simulink model "mpc_payload"  (R2020a)
settings: Solver=ode3  StartTime=0.0  StopTime=200  FixedStep=Ts_sim  RelTol=1e-3
InitFcn:
  | initialise_ros_iris_payload
values from neighbouring files (symbols this model uses):
  A_mpc = A_havok    [initialize_mpc_iris_no_load.m]    (also in initialize_mpc_iris_payload.m = [zeros( size(A_mpc,1), num_axis ), A_mpc])
  enable_mpc_control = 1    [initialise_ros_iris_payload.m]
  max_vel_xy = 5    [initialise_iris_gains.m]
  max_vel_z_down = 5    [initialise_iris_gains.m]
  max_vel_z_up = 5    [initialise_iris_gains.m]
  mpc_step_time = 2    [initialise_ros_iris_payload.m]
  MPC_XY_VEL_D_ACC = 0.2    [initialise_iris_gains.m]
  MPC_XY_VEL_I_ACC = 0.4    [initialise_iris_gains.m]
  MPC_XY_VEL_P_ACC = 1.8    [initialise_iris_gains.m]
  MPC_Z_VEL_D_ACC = 0    [initialise_iris_gains.m]
  MPC_Z_VEL_I_ACC = 2    [initialise_iris_gains.m]
  MPC_Z_VEL_P_ACC = 4    [initialise_iris_gains.m]
  Ts_pos_control = 0.01    [initialise_ros_iris_payload.m]
  vel_step_size = 1    [initialise_ros_iris_payload.m]
  y_ext_0 = zeros(q*ny, 1)    [initialize_mpc_iris_no_load.m]    (also in initialize_mpc_iris_payload.m)
undefined symbols (not defined in the file or in its folder): DiscIntNeverNeededParam, MPC_ACC_DOWN_MAX, MPC_ACC_HOR_MAX, MPC_ACC_UP_MAX, ny, q, q_int_lim, u_bar, vel_filt_denom, vel_filt_num, X, Y, Z
libraries: robotlib x6, simulink x3, robotgazebolib x1, mpclib x1
settings Model: Creator=esl  LastModifiedBy=murray
settings SolverCC: MinimalZcImpactIntegration=on
settings OptimizationCC: DefaultParameterBehavior=Inlined  GainParamInheritBuiltInType=on  UseFloatMulNetSlope=on  InlineInvariantSignals=on  EnhancedBackFolding=on  PassReuseOutputArgsAs=Individual arguments  ZeroExternalMemoryAtStartup=off  ZeroInternalMemoryAtStartup=off  EfficientFloat2IntCast=on  MaxStackSize=64  OptimizeBlockOrder=speed  DifferentSizesBufferReuse=on  OptimizationCustomize=off  EfficientTunableParamExpr=on
settings DebuggingCC: ReadBeforeWriteMsg=DisableAll  WriteAfterWriteMsg=DisableAll  WriteAfterReadMsg=DisableAll  MultiTaskDSMMsg=none  ParameterTunabilityLossMsg=error  SFMachineParentedDataDiag=error
settings HardwareCC: ProdBitPerPointer=32  ProdBitPerSizeT=32  ProdBitPerPtrDiffT=32  ProdLargestAtomicInteger=Long  ProdLargestAtomicFloat=Double  ProdWordSize=32  ProdHWDeviceType=ARM Compatible->ARM Cortex  UseEmbeddedCoderFeatures=off
settings ModelReferenceCC: UpdateModelReferenceTargets=IfOutOfDate
settings SFSimCC: SFSimEcho=off  MATLABDynamicMemAlloc=off
settings RTWCC: SystemTargetFile=ert.tlc  HardwareBoard=Robot Operating System (ROS)  TemplateMakefile=ert_default_tmf  Toolchain=Catkin  BuildConfiguration=Faster Runs  TargetLang=C++
settings CodeAppCC: ForceParamTrailComments=on  IgnoreCustomStorageClasses=off  OperatorAnnotations=on  SimulinkDataObjDesc=on  SFDataObjDesc=on  InsertBlockDesc=on
settings ERTTargetCC: SupportNonFinite=off  SupportNonInlinedSFcns=on  ERTCustomFileTemplate=rostime_codertarget_file_process.tlc

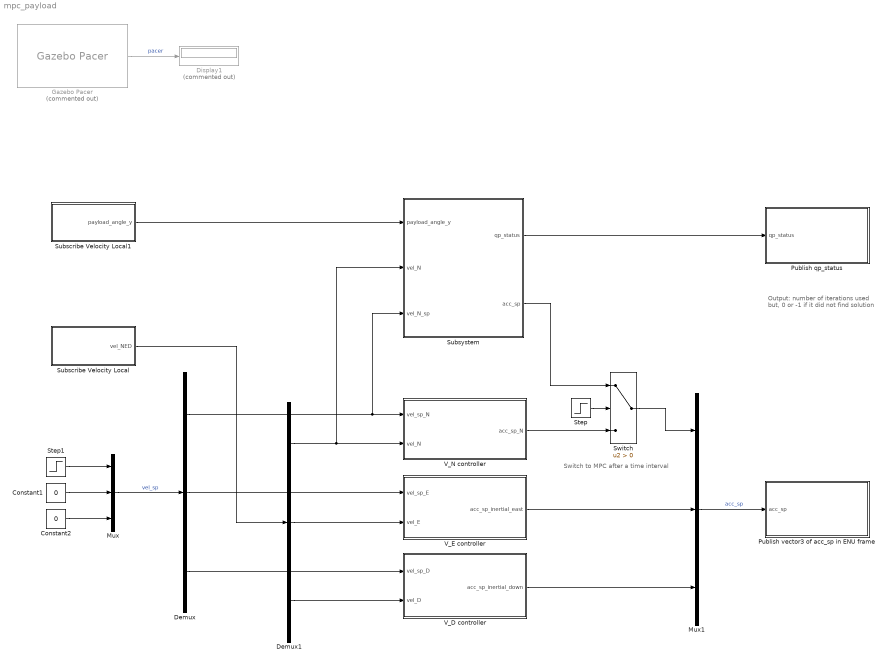
== system mpc_payload ==
  note: Output: number of iterations used
      | but, 0 or -1 if it did not find solution
  note: Switch to MPC after a time interval
  Constant1 : Constant  Value=0
  Constant2 : Constant  Value=0
  Demux : Demux  Outputs=3
  Demux1 : Demux  Outputs=3
  Display1 : Display  Commented=on
  Gazebo Pacer : robotgazebolib/Gazebo Pacer  Commented=on  ResetBehavior=Reset Gazebo simulation time  SampleTime=0.004
      settings: SourceProductBaseCode=RO
  Mux : Mux  Inputs=3
  Mux1 : Mux  Inputs=3
  Publish qp_status : Subsystem
  Publish vector3 of acc_sp in ENU frame : Subsystem
  Step : Step  Time=mpc_step_time  After=enable_mpc_control  SampleTime=0
  Step1 : Step  Time=mpc_step_time  After=vel_step_size  SampleTime=0
  Subscribe Velocity Local : Subsystem
  Subscribe Velocity Local1 : Subsystem
  Subsystem : Subsystem
  Switch : Switch  Criteria=u2 > Threshold
  V_D controller : Subsystem
  V_E controller : Subsystem
  V_N controller : Subsystem
  wires:
  Gazebo Pacer/1 -> Display1/1  "pacer"
  V_D controller/1(acc_sp_inertial_down) -> Mux1/3
  V_E controller/1(acc_sp_inertial_east) -> Mux1/2
  Mux1/1 -> Publish vector3 of acc_sp in ENU frame/1(acc_sp)  "acc_sp"
  Subsystem/2(acc_sp) -> Switch/1
  Mux/1 -> Demux/1  "vel_sp"
  Demux/2 -> V_E controller/1(vel_sp_E)
  Demux/3 -> V_D controller/1(vel_sp_D)
  Demux1/2 -> V_E controller/2(vel_E)
  Demux1/3 -> V_D controller/2(vel_D)
  Subscribe Velocity Local/1(vel_NED) -> Demux1/1
  Demux/1 -> Subsystem/3(vel_N_sp), V_N controller/1(vel_sp_N)
  Demux1/1 -> Subsystem/2(vel_N), V_N controller/2(vel_N)
  Step/1 -> Switch/2
  V_N controller/1(acc_sp_N) -> Switch/3
  Switch/1 -> Mux1/1
  Step1/1 -> Mux/1
  Constant1/1 -> Mux/2
  Constant2/1 -> Mux/3
  Subscribe Velocity Local1/1(payload_angle_y) -> Subsystem/1(payload_angle_y)
  Subsystem/1(qp_status) -> Publish qp_status/1(qp_status)

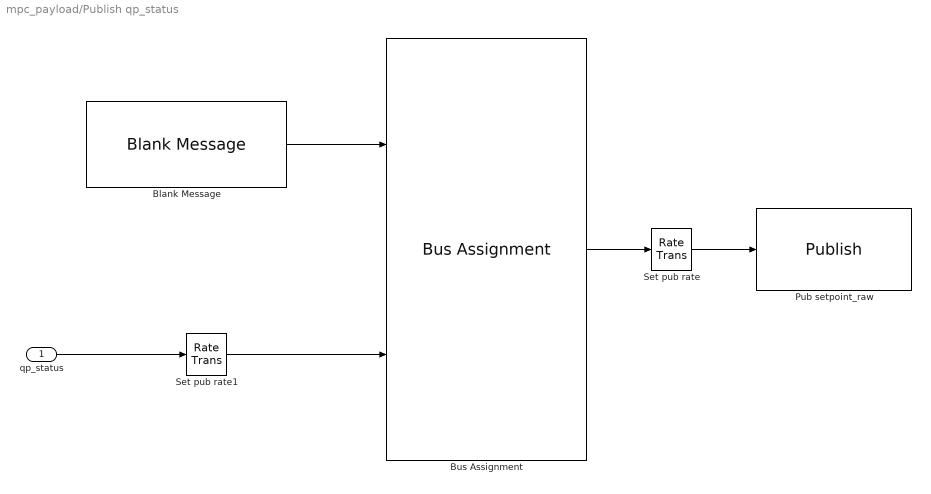
== system mpc_payload/Publish qp_status ==
  qp_status : Inport
  Blank Message : robotlib/Blank Message  messageClass=Message  entityType=std_msgs/Float64  messageType=std_msgs/Float64  SampleTime=inf
  Bus Assignment : BusAssignment  AssignedSignals=Data
  Pub setpoint_raw : robotlib/Publish  topicSource=Specify your own  topic=/simulink/qp_status  messageType=std_msgs/Float64  messageQueueLength=1
  Set pub rate : RateTransition  OutPortSampleTime=Ts_publish
  Set pub rate1 : RateTransition  OutPortSampleTime=Ts_publish
  wires:
  Set pub rate/1 -> Pub setpoint_raw/1
  Bus Assignment/1 -> Set pub rate/1
  Blank Message/1 -> Bus Assignment/1
  qp_status/1 -> Set pub rate1/1
  Set pub rate1/1 -> Bus Assignment/2

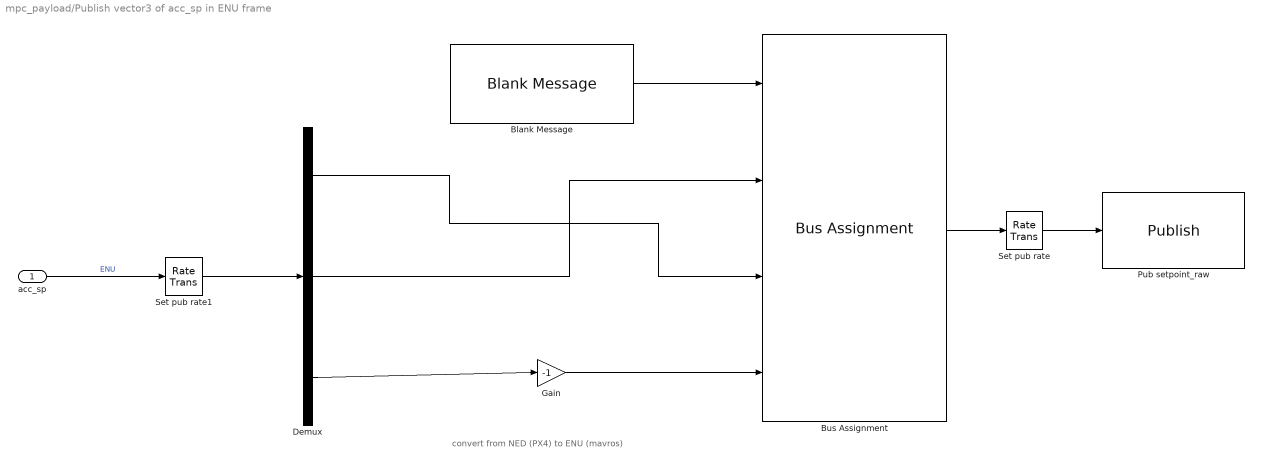
== system mpc_payload/Publish vector3 of acc_sp in ENU frame ==
  note: convert from NED (PX4) to ENU (mavros)
  acc_sp : Inport
  Blank Message : robotlib/Blank Message  messageClass=Message  entityType=geometry_msgs/Vector3  messageType=geometry_msgs/Vector3  SampleTime=inf
  Bus Assignment : BusAssignment  AssignedSignals=X,Y,Z
  Demux : Demux  Outputs=3
  Gain : Gain  Gain=-1
  Pub setpoint_raw : robotlib/Publish  topicSource=Specify your own  topic=/simulink/acc_sp  messageType=geometry_msgs/Vector3  messageQueueLength=1
  Set pub rate : RateTransition  OutPortSampleTime=Ts_publish
  Set pub rate1 : RateTransition  OutPortSampleTime=Ts_publish
  wires:
  Set pub rate/1 -> Pub setpoint_raw/1
  Bus Assignment/1 -> Set pub rate/1
  Blank Message/1 -> Bus Assignment/1
  Demux/1 -> Bus Assignment/3
  Demux/2 -> Bus Assignment/2
  Demux/3 -> Gain/1
  Gain/1 -> Bus Assignment/4
  acc_sp/1 -> Set pub rate1/1  "ENU"
  Set pub rate1/1 -> Demux/1

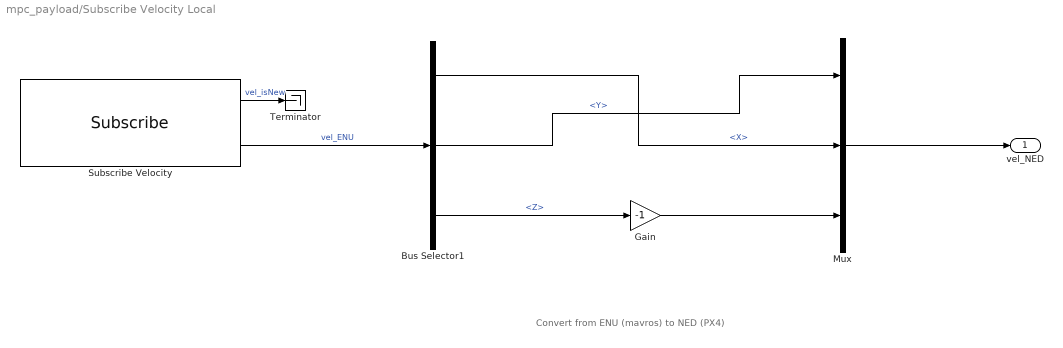
== system mpc_payload/Subscribe Velocity Local ==
  note: Convert from ENU (mavros) to NED (PX4)
  Bus Selector1 : BusSelector  OutputSignals=Twist.Linear.X,Twist.Linear.Y,Twist.Linear.Z
  Gain : Gain  Gain=-1
  Mux : Mux  Inputs=3
  Subscribe Velocity : robotlib/Subscribe  topicSource=Select from ROS network  topic=/mavros/local_position/velocity_local  messageType=geometry_msgs/TwistStamped  sampleTime=Ts_sub  messageQueueLength=1
  Terminator : Terminator
  vel_NED : Outport
  wires:
  Subscribe Velocity/1 -> Terminator/1  "vel_isNew"
  Subscribe Velocity/2 -> Bus Selector1/1  "vel_ENU"
  Mux/1 -> vel_NED/1
  Bus Selector1/1 -> Mux/2  "<X>"
  Bus Selector1/2 -> Mux/1  "<Y>"
  Bus Selector1/3 -> Gain/1  "<Z>"
  Gain/1 -> Mux/3

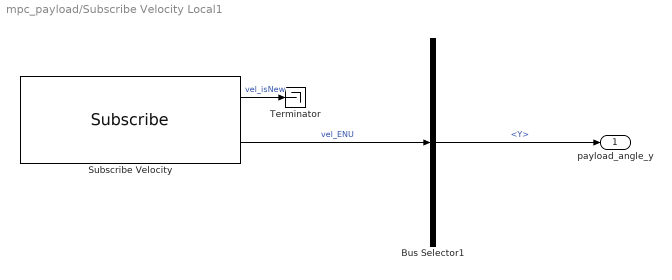
== system mpc_payload/Subscribe Velocity Local1 ==
  Bus Selector1 : BusSelector  OutputSignals=Y
  Subscribe Velocity : robotlib/Subscribe  topicSource=Select from ROS network  topic=/simulink/payload_angles  messageType=geometry_msgs/Vector3  sampleTime=Ts_sub  messageQueueLength=1
  Terminator : Terminator
  payload_angle_y : Outport
  wires:
  Subscribe Velocity/1 -> Terminator/1  "vel_isNew"
  Subscribe Velocity/2 -> Bus Selector1/1  "vel_ENU"
  Bus Selector1/1 -> payload_angle_y/1  "<Y>"

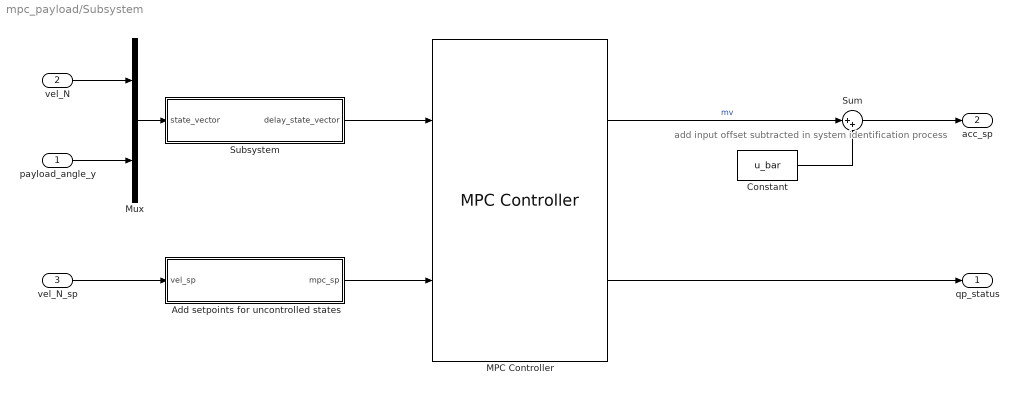
== system mpc_payload/Subsystem ==
  note: add input offset subtracted in system identification process
  payload_angle_y : Inport
  vel_N : Inport  Port=2
  vel_N_sp : Inport  Port=3
  Add setpoints for uncontrolled states : Subsystem
  Constant : Constant  Value=u_bar
  MPC Controller : mpclib/MPC Controller  SCDEnableBlockLinearizationSpecification=on  mpcobj=mpc_iris_payload  is_multiple=0  enable_value=0  return_u0=off  updateMPCinCallerWorkspace=on  md_inport=off  mv_inport=off  uref_inport=off  return_cost=off  return_mvseq=off  return_qpstatus=on  return_xseq=off  return_state=off  return_ovseq=off  state_inport=off  umin_inport=off  umax_inport=off  ymin_inport=off  ymax_inport=off  cc_inport=off  ywt_inport=off  uwt_inport=off  duwt_inport=off  rhoeps_inport=off  pm_inport=off  MaximumP=10  HorizonChoice=FixedHorizon  n_ts=0.03  n_p=166  n_mv=1  n_md=0  n_ud=0  n_mo=140  n_uo=1  BlockDataType=double  SampleTimeInherited=off  switch_inport=off
  Mux : Mux  Inputs=2
  Subsystem : Subsystem
  Sum : Sum  Inputs=|++
  qp_status : Outport  OutDataTypeStr=double  PortDimensions=nu
  acc_sp : Outport  Port=2  OutDataTypeStr=double  PortDimensions=nu
  wires:
  Sum/1 -> acc_sp/1
  MPC Controller/1 -> Sum/1  "mv"
  Constant/1 -> Sum/2
  Subsystem/1(delay_state_vector) -> MPC Controller/1
  Add setpoints for uncontrolled states/1(mpc_sp) -> MPC Controller/2
  vel_N_sp/1 -> Add setpoints for uncontrolled states/1(vel_sp)
  Mux/1 -> Subsystem/1(state_vector)
  vel_N/1 -> Mux/1
  payload_angle_y/1 -> Mux/2
  MPC Controller/2 -> qp_status/1

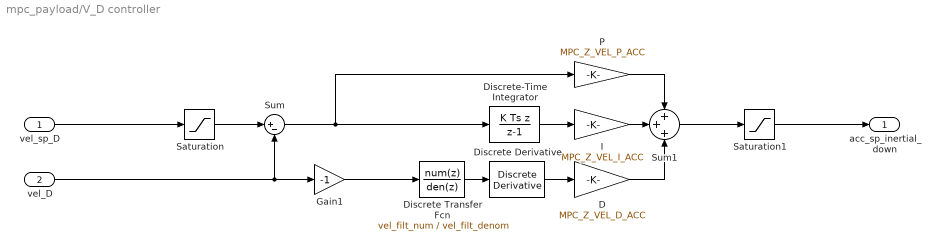
== system mpc_payload/V_D controller ==
  vel_sp_D : Inport  SampleTime=Ts_pos_control
  vel_D : Inport  Port=2  SampleTime=Ts_pos_control
  D : Gain  Gain=MPC_Z_VEL_D_ACC
  Discrete Transfer Fcn : DiscreteTransferFcn  Numerator=vel_filt_num  Denominator=vel_filt_denom
  Discrete Derivative : simulink/Discrete/Discrete Derivative  gainval=1  ICPrevScaledInput=0.0  OutMin=[]  OutMax=[]  OutDataType=fixdt(1, 16)  OutScaling=2^-10  DoSatur=off
  Discrete-Time Integrator : DiscreteIntegrator  IntegratorMethod=Integration: Backward Euler  gainval=1  SampleTime=-1  UpperSaturationLimit=q_int_lim  LowerSaturationLimit=-q_int_lim  ICPrevOutput=DiscIntNeverNeededParam  ICPrevScaledInput=DiscIntNeverNeededParam
  Gain1 : Gain  Gain=-1
  I : Gain  Gain=MPC_Z_VEL_I_ACC
  P : Gain  Gain=MPC_Z_VEL_P_ACC
  Saturation : Saturate  UpperLimit=max_vel_z_up  LowerLimit=-abs(max_vel_z_down)
  Saturation1 : Saturate  UpperLimit=MPC_ACC_UP_MAX  LowerLimit=-MPC_ACC_DOWN_MAX
  Sum : Sum  Inputs=|+-
  Sum1 : Sum  Inputs=+++
  acc_sp_inertial_down : Outport  VectorParamsAs1DForOutWhenUnconnected=off
  wires:
  vel_sp_D/1 -> Saturation/1
  Discrete Derivative/1 -> D/1
  I/1 -> Sum1/2
  D/1 -> Sum1/3
  vel_D/1 -> Gain1/1, Sum/2
  P/1 -> Sum1/1
  Sum/1 -> Discrete-Time Integrator/1, P/1
  Discrete Transfer Fcn/1 -> Discrete Derivative/1
  Saturation/1 -> Sum/1
  Discrete-Time Integrator/1 -> I/1
  Sum1/1 -> Saturation1/1
  Gain1/1 -> Discrete Transfer Fcn/1
  Saturation1/1 -> acc_sp_inertial_down/1

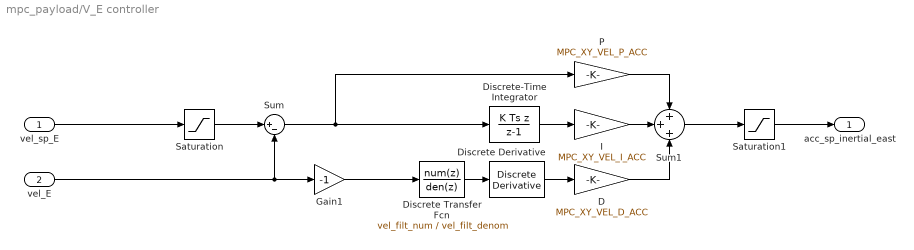
== system mpc_payload/V_E controller ==
  vel_sp_E : Inport  SampleTime=Ts_pos_control
  vel_E : Inport  Port=2  SampleTime=Ts_pos_control
  D : Gain  Gain=MPC_XY_VEL_D_ACC
  Discrete Transfer Fcn : DiscreteTransferFcn  Numerator=vel_filt_num  Denominator=vel_filt_denom
  Discrete Derivative : simulink/Discrete/Discrete Derivative  gainval=1  ICPrevScaledInput=0.0  OutMin=[]  OutMax=[]  OutDataType=fixdt(1, 16)  OutScaling=2^-10  DoSatur=off
  Discrete-Time Integrator : DiscreteIntegrator  IntegratorMethod=Integration: Backward Euler  gainval=1  SampleTime=-1  UpperSaturationLimit=q_int_lim  LowerSaturationLimit=-q_int_lim  ICPrevOutput=DiscIntNeverNeededParam  ICPrevScaledInput=DiscIntNeverNeededParam
  Gain1 : Gain  Gain=-1
  I : Gain  Gain=MPC_XY_VEL_I_ACC
  P : Gain  Gain=MPC_XY_VEL_P_ACC
  Saturation : Saturate  UpperLimit=max_vel_xy  LowerLimit=-max_vel_xy
  Saturation1 : Saturate  UpperLimit=MPC_ACC_HOR_MAX  LowerLimit=-MPC_ACC_HOR_MAX
  Sum : Sum  Inputs=|+-
  Sum1 : Sum  Inputs=+++
  acc_sp_inertial_east : Outport  VectorParamsAs1DForOutWhenUnconnected=off
  wires:
  vel_E/1 -> Gain1/1, Sum/2
  Discrete-Time Integrator/1 -> I/1
  Sum/1 -> Discrete-Time Integrator/1, P/1
  vel_sp_E/1 -> Saturation/1
  Sum1/1 -> Saturation1/1
  Saturation/1 -> Sum/1
  Discrete Transfer Fcn/1 -> Discrete Derivative/1
  Discrete Derivative/1 -> D/1
  I/1 -> Sum1/2
  Gain1/1 -> Discrete Transfer Fcn/1
  P/1 -> Sum1/1
  D/1 -> Sum1/3
  Saturation1/1 -> acc_sp_inertial_east/1

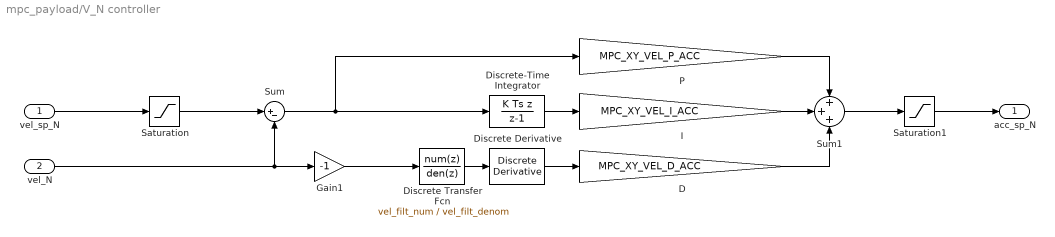
== system mpc_payload/V_N controller ==
  vel_sp_N : Inport  SampleTime=Ts_pos_control
  vel_N : Inport  Port=2  SampleTime=Ts_pos_control
  D : Gain  Gain=MPC_XY_VEL_D_ACC
  Discrete Transfer Fcn : DiscreteTransferFcn  Numerator=vel_filt_num  Denominator=vel_filt_denom
  Discrete Derivative : simulink/Discrete/Discrete Derivative  gainval=1  ICPrevScaledInput=0.0  OutMin=[]  OutMax=[]  OutDataType=fixdt(1, 16)  OutScaling=2^-10  DoSatur=off
  Discrete-Time Integrator : DiscreteIntegrator  IntegratorMethod=Integration: Backward Euler  gainval=1  SampleTime=-1  UpperSaturationLimit=max_vel_xy  LowerSaturationLimit=-max_vel_xy  ICPrevOutput=DiscIntNeverNeededParam  ICPrevScaledInput=DiscIntNeverNeededParam
  Gain1 : Gain  Gain=-1
  I : Gain  Gain=MPC_XY_VEL_I_ACC
  P : Gain  Gain=MPC_XY_VEL_P_ACC
  Saturation : Saturate  UpperLimit=max_vel_xy  LowerLimit=-max_vel_xy
  Saturation1 : Saturate  UpperLimit=MPC_ACC_HOR_MAX  LowerLimit=-MPC_ACC_HOR_MAX
  Sum : Sum  Inputs=|+-
  Sum1 : Sum  Inputs=+++
  acc_sp_N : Outport  VectorParamsAs1DForOutWhenUnconnected=off
  wires:
  vel_N/1 -> Gain1/1, Sum/2
  vel_sp_N/1 -> Saturation/1
  I/1 -> Sum1/2
  Sum/1 -> Discrete-Time Integrator/1, P/1
  P/1 -> Sum1/1
  Sum1/1 -> Saturation1/1
  Discrete Derivative/1 -> D/1
  Discrete Transfer Fcn/1 -> Discrete Derivative/1
  D/1 -> Sum1/3
  Saturation/1 -> Sum/1
  Gain1/1 -> Discrete Transfer Fcn/1
  Discrete-Time Integrator/1 -> I/1
  Saturation1/1 -> acc_sp_N/1

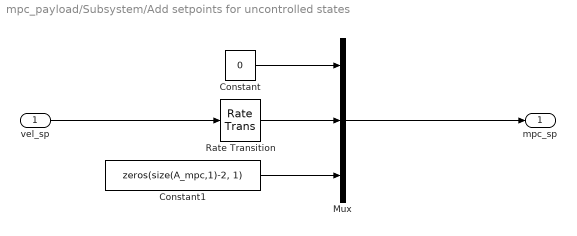
== system mpc_payload/Subsystem/Add setpoints for uncontrolled states ==
  vel_sp : Inport
  Constant : Constant  Value=0
  Constant1 : Constant  Value=zeros(size(A_mpc,1)-2, 1)
  Mux : Mux  Inputs=3
  Rate Transition : RateTransition  Deterministic=off  OutPortSampleTime=Ts_mpc
  mpc_sp : Outport
  wires:
  Constant1/1 -> Mux/3
  vel_sp/1 -> Rate Transition/1
  Mux/1 -> mpc_sp/1
  Rate Transition/1 -> Mux/2
  Constant/1 -> Mux/1

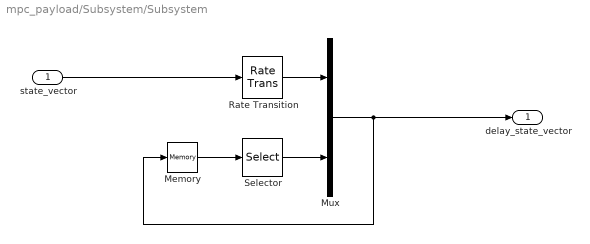
== system mpc_payload/Subsystem/Subsystem ==
  state_vector : Inport
  Memory : Memory  InitialCondition=y_ext_0
  Mux : Mux  Inputs=2
  Rate Transition : RateTransition  OutPortSampleTime=Ts_mpc
  Selector : Selector  IndexMode=Zero-based  InputPortWidth=ny*q  IndexOptions=Index vector (dialog)  Indices=0:ny*(q-1)-1  OutputSizes=1
  delay_state_vector : Outport
  wires:
  Memory/1 -> Selector/1
  state_vector/1 -> Rate Transition/1
  Mux/1 -> Memory/1, delay_state_vector/1
  Selector/1 -> Mux/2
  Rate Transition/1 -> Mux/1
